simulink model "pi_seqIface"  (R2018b)
settings: Solver=FixedStepDiscrete  StartTime=0.0  StopTime=10.0  RelTol=1e-3
undefined symbols (not defined in the file): boolAliasMember, boolMember, choiceAliasesMember, choiceBuiltInMember, choiceOfFixedSizeSeqOfsMember, choiceOfVarSizeSeqOfsMember, enumAliasMember, enumMember, ia5StringFixedSizeAliasMember, ia5StringFixedSizeMember, ia5StringVarSizeAliasMember, ia5StringVarSizeMember, integerAliasMember, integerMember, octetStringFixedSizeAliasMember, octetStringFixedSizeMember, octetStringVarSizeAliasMember, octetStringVarSizeMember, realAliasMember, realMember
settings Model: Creator=matlab  LastModifiedBy=matlab
settings DataIOCC: SaveOutput=off  SignalLogging=off  SaveTime=off
settings OptimizationCC: DefaultParameterBehavior=Inlined  EnhancedBackFolding=on  PassReuseOutputArgsAs=Individual arguments  OptimizeBlockOrder=speed  DifferentSizesBufferReuse=on  OptimizationCustomize=off
settings DebuggingCC: ParameterTunabilityLossMsg=error
settings SFSimCC: MATLABDynamicMemAlloc=off
settings RTWCC: SystemTargetFile=ert.tlc  TemplateMakefile=ert_default_tmf  PostCodeGenCommand=packNGo(buildInfo);  GenerateReport=on  IncludeHyperlinkInReport=on  LaunchReport=on  GenerateTraceInfo=on  GenerateTraceReport=on  GenerateTraceReportSl=on  GenerateTraceReportSf=on  GenerateTraceReportEml=on
settings CodeAppCC: ForceParamTrailComments=on  IgnoreCustomStorageClasses=off  OperatorAnnotations=on  SimulinkDataObjDesc=on  SFDataObjDesc=on  InsertBlockDesc=on
settings ERTTargetCC: TargetLangStandard=C99 (ISO)  GenerateSampleERTMain=on  InlinedParameterPlacement=NonHierarchical  ERTCustomFileTemplate=example_file_process.tlc

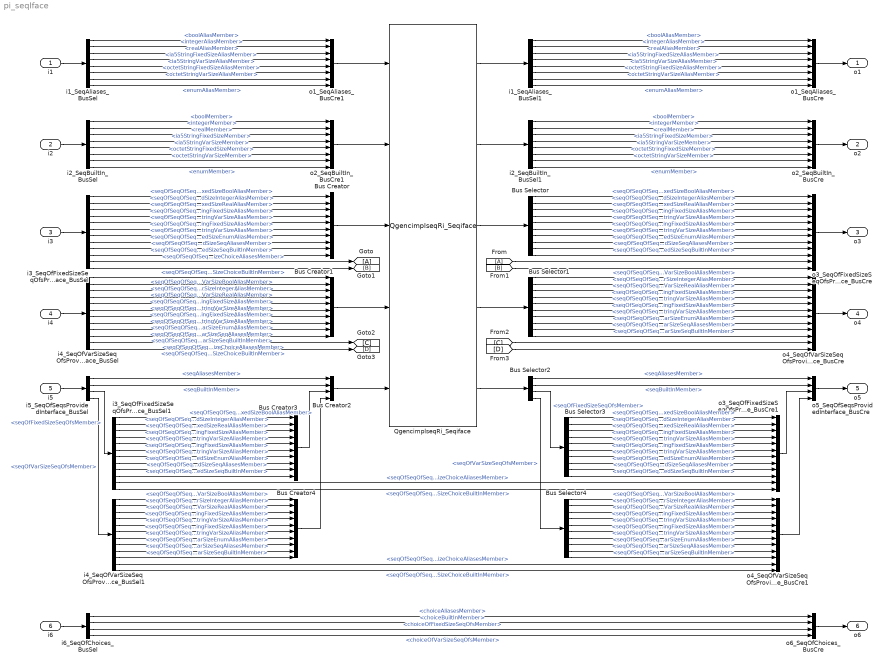
== system pi_seqIface ==
  i1 : Inport  OutDataTypeStr=Bus: SeqAliases  BusOutputAsStruct=on
  i2 : Inport  Port=2  OutDataTypeStr=Bus: SeqBuiltIn  BusOutputAsStruct=on
  i3 : Inport  Port=3  OutDataTypeStr=Bus: SeqOfFixedSizeSeqOfsProvidedInterface  BusOutputAsStruct=on
  i4 : Inport  Port=4  OutDataTypeStr=Bus: SeqOfVarSizeSeqOfsProvidedInterface  BusOutputAsStruct=on
  i5 : Inport  Port=5  OutDataTypeStr=Bus: SeqOfSeqsProvidedInterface  BusOutputAsStruct=on
  i6 : Inport  Port=6  OutDataTypeStr=Bus: SeqOfChoices  BusOutputAsStruct=on
  Bus Creator : BusCreator  Inputs=10  OutDataTypeStr=Bus: SeqOfFixedSizeSeqOfsRequiredInterface  NonVirtualBus=on
  Bus Creator1 : BusCreator  Inputs=10  OutDataTypeStr=Bus: SeqOfVarSizeSeqOfsRequiredInterface  NonVirtualBus=on
  Bus Creator2 : BusCreator  Inputs=4  OutDataTypeStr=Bus: SeqOfSeqsRequiredInterface  NonVirtualBus=on
  Bus Creator3 : BusCreator  Inputs=10  OutDataTypeStr=Bus: SeqOfFixedSizeSeqOfsRequiredInterface  NonVirtualBus=on
  Bus Creator4 : BusCreator  Inputs=10  OutDataTypeStr=Bus: SeqOfVarSizeSeqOfsRequiredInterface  NonVirtualBus=on
  Bus Selector : BusSelector  OutputSignals=seqOfSeqOfSeqOfFixedSizeBoolAliasMember,seqOfSeqOfSeqOfFixedSizeIntegerAliasMember,seqOfSeqOfSeqOfFixedSizeRealAliasMember,seqOfSeqOfSeqOfFixedSizeIA5StringFixedSizeAliasMember,seqOfSeqOfSeqOfFixedSizeIA5StringVarSizeAliasMember,seqOfSeqOfSeqOfFixedSizeOctetStringFixedSizeAliasMember,seqOfSeqOfSeqOfFixedSizeOctetStringVarSizeAliasMember,seqOfSeqOfSeqOfFixedSizeEnumAliasMember,seqOfSeqOfSeqOfFixedSizeSeqAliasesMember,seqOfSeqOfSeqOfFixedSizeSeqBuiltInMember
  Bus Selector1 : BusSelector  OutputSignals=seqOfSeqOfSeqOfVarSizeBoolAliasMember,seqOfSeqOfSeqOfVarSizeIntegerAliasMember,seqOfSeqOfSeqOfVarSizeRealAliasMember,seqOfSeqOfSeqOfVarSizeIA5StringFixedSizeAliasMember,seqOfSeqOfSeqOfVarSizeIA5StringVarSizeAliasMember,seqOfSeqOfSeqOfVarSizeOctetStringFixedSizeAliasMember,seqOfSeqOfSeqOfVarSizeOctetStringVarSizeAliasMember,seqOfSeqOfSeqOfVarSizeEnumAliasMember,seqOfSeqOfSeqOfVarSizeSeqAliasesMember,seqOfSeqOfSeqOfVarSizeSeqBuiltInMember
  Bus Selector2 : BusSelector  OutputSignals=seqAliasesMember,seqBuiltInMember,seqOfFixedSizeSeqOfsMember,seqOfVarSizeSeqOfsMember
  Bus Selector3 : BusSelector  OutputSignals=seqOfSeqOfSeqOfFixedSizeBoolAliasMember,seqOfSeqOfSeqOfFixedSizeIntegerAliasMember,seqOfSeqOfSeqOfFixedSizeRealAliasMember,seqOfSeqOfSeqOfFixedSizeIA5StringFixedSizeAliasMember,seqOfSeqOfSeqOfFixedSizeIA5StringVarSizeAliasMember,seqOfSeqOfSeqOfFixedSizeOctetStringFixedSizeAliasMember,seqOfSeqOfSeqOfFixedSizeOctetStringVarSizeAliasMember,seqOfSeqOfSeqOfFixedSizeEnumAliasMember,seqOfSeqOfSeqOfFixedSizeSeqAliasesMember,seqOfSeqOfSeqOfFixedSizeSeqBuiltInMember
  Bus Selector4 : BusSelector  OutputSignals=seqOfSeqOfSeqOfVarSizeBoolAliasMember,seqOfSeqOfSeqOfVarSizeIntegerAliasMember,seqOfSeqOfSeqOfVarSizeRealAliasMember,seqOfSeqOfSeqOfVarSizeIA5StringFixedSizeAliasMember,seqOfSeqOfSeqOfVarSizeIA5StringVarSizeAliasMember,seqOfSeqOfSeqOfVarSizeOctetStringFixedSizeAliasMember,seqOfSeqOfSeqOfVarSizeOctetStringVarSizeAliasMember,seqOfSeqOfSeqOfVarSizeEnumAliasMember,seqOfSeqOfSeqOfVarSizeSeqAliasesMember,seqOfSeqOfSeqOfVarSizeSeqBuiltInMember
  QgencimplseqRi_Seqiface : S-Function  FunctionName=QgencimplseqRi_Seqiface  SFunctionDeploymentMode=off  EnableBusSupport=off  mask(Legacy Function){SFunctionSpec=void qgencimplseq_RI_ri_seqIface(SeqAliases u1[1], SeqBuiltIn u2[1], SeqOfFixedSizeSeqOfsRequiredInterface u3[1], SeqOfVarSizeSeqOfsRequiredInterface u4[1], SeqOfSeqsRequiredInterface u5[1], SeqAliases y1[1], SeqBuiltIn y2[1], SeqOfFixedSizeSeqOfsRequiredInterface y3[1], SeqOfVarSizeSeqOfsRequiredInterface y4[1], SeqOfSeqsRequiredInterface y5[1]), ShowSpec=off}
      mask prompts: ShowSpec "Display function specification"
      mask help:
      | This block allows you to call the legacy functions specified by the following Legacy Code Tool definition:
      | def.SFunctionName = 'QgencimplseqRi_Seqiface';
      | def.OutputFcnSpec = 'void qgencimplseq_RI_ri_seqIface(SeqAliases u1[1], SeqBuiltIn u2[1], SeqOfFixedSizeSeqOfsRequiredInterface u3[1], SeqOfVarSizeSeqOfsRequiredInterface u4[1], SeqOfSeqsRequiredInterface u5[1], SeqAliases y1[1], SeqBuiltIn y2[1], SeqOfFixedSizeSeqOfsRequiredInterface y3[1], SeqOfVarSizeSeqOfsRequiredInterface y4[1], SeqOfSeqsRequiredInterface y5[1])';
      | def.HeaderFiles = {'qgencimplseq_invoke_ri.h'};
      | def.SourceFiles = {'qgencimplseq_invoke_ri.c'};
      | def.IncPaths = {'..\..\..\dataview\C'};
      mask Help: <p>This block was generated automatically by the Legacy Code Tool. For detailed help on this tool, call<a href="matlab:legacy_code('help')"> legacy_code('help')</a>.</p>
      mask Callback ShowSpec:
      | if strcmp(get_param(gcbh, 'ShowSpec'), 'on')
      |   set_param(gcbh, 'MaskDisplay', sprintf('fprintf(''%s'');', get_param(gcbh, 'SFunctionSpec')));
      | else
      |   set_param(gcbh, 'MaskDisplay', sprintf('fprintf(''%s'');', get_param(gcbh, 'FunctionName')));
      | end
      mask Display: fprintf('QgencimplseqRi_Seqiface');
  i1_SeqAliases_BusSel : BusSelector  OutputSignals=boolAliasMember,integerAliasMember,realAliasMember,ia5StringFixedSizeAliasMember,ia5StringVarSizeAliasMember,octetStringFixedSizeAliasMember,octetStringVarSizeAliasMember,enumAliasMember
  i1_SeqAliases_BusSel1 : BusSelector  OutputSignals=boolAliasMember,integerAliasMember,realAliasMember,ia5StringFixedSizeAliasMember,ia5StringVarSizeAliasMember,octetStringFixedSizeAliasMember,octetStringVarSizeAliasMember,enumAliasMember
  i2_SeqBuiltIn_BusSel : BusSelector  OutputSignals=boolMember,integerMember,realMember,ia5StringFixedSizeMember,ia5StringVarSizeMember,octetStringFixedSizeMember,octetStringVarSizeMember,enumMember
  i2_SeqBuiltIn_BusSel1 : BusSelector  OutputSignals=boolMember,integerMember,realMember,ia5StringFixedSizeMember,ia5StringVarSizeMember,octetStringFixedSizeMember,octetStringVarSizeMember,enumMember
  i3_SeqOfFixedSizeSeqOfsProvidedInterface_BusSel : BusSelector  OutputSignals=seqOfSeqOfSeqOfFixedSizeBoolAliasMember,seqOfSeqOfSeqOfFixedSizeIntegerAliasMember,seqOfSeqOfSeqOfFixedSizeRealAliasMember,seqOfSeqOfSeqOfFixedSizeIA5StringFixedSizeAliasMember,seqOfSeqOfSeqOfFixedSizeIA5StringVarSizeAliasMember,seqOfSeqOfSeqOfFixedSizeOctetStringFixedSizeAliasMember,seqOfSeqOfSeqOfFixedSizeOctetStringVarSizeAliasMember,seqOfSeqOfSeqOfFixedSizeEnumAliasMember,seqOfSeqOfSeqOfFixedSizeSeqAliasesMember,seqOfSeqOfSeqOfFixedSizeSeqBuiltInMember,seqOfSeqOfSeqOfFixedSizeChoiceAliasesMember,seqOfSeqOfSeqOfFixedSizeChoiceBuiltInMember
  i3_SeqOfFixedSizeSeqOfsProvidedInterface_BusSel1 : BusSelector  OutputSignals=seqOfSeqOfSeqOfFixedSizeBoolAliasMember,seqOfSeqOfSeqOfFixedSizeIntegerAliasMember,seqOfSeqOfSeqOfFixedSizeRealAliasMember,seqOfSeqOfSeqOfFixedSizeIA5StringFixedSizeAliasMember,seqOfSeqOfSeqOfFixedSizeIA5StringVarSizeAliasMember,seqOfSeqOfSeqOfFixedSizeOctetStringFixedSizeAliasMember,seqOfSeqOfSeqOfFixedSizeOctetStringVarSizeAliasMember,seqOfSeqOfSeqOfFixedSizeEnumAliasMember,seqOfSeqOfSeqOfFixedSizeSeqAliasesMember,seqOfSeqOfSeqOfFixedSizeSeqBuiltInMember,seqOfSeqOfSeqOfFixedSizeChoiceAliasesMember,seqOfSeqOfSeqOfFixedSizeChoiceBuiltInMember
  i4_SeqOfVarSizeSeqOfsProvidedInterface_BusSel : BusSelector  OutputSignals=seqOfSeqOfSeqOfVarSizeBoolAliasMember,seqOfSeqOfSeqOfVarSizeIntegerAliasMember,seqOfSeqOfSeqOfVarSizeRealAliasMember,seqOfSeqOfSeqOfVarSizeIA5StringFixedSizeAliasMember,seqOfSeqOfSeqOfVarSizeIA5StringVarSizeAliasMember,seqOfSeqOfSeqOfVarSizeOctetStringFixedSizeAliasMember,seqOfSeqOfSeqOfVarSizeOctetStringVarSizeAliasMember,seqOfSeqOfSeqOfVarSizeEnumAliasMember,seqOfSeqOfSeqOfVarSizeSeqAliasesMember,seqOfSeqOfSeqOfVarSizeSeqBuiltInMember,seqOfSeqOfSeqOfVarSizeChoiceAliasesMember,seqOfSeqOfSeqOfVarSizeChoiceBuiltInMember
  i4_SeqOfVarSizeSeqOfsProvidedInterface_BusSel1 : BusSelector  OutputSignals=seqOfSeqOfSeqOfVarSizeBoolAliasMember,seqOfSeqOfSeqOfVarSizeIntegerAliasMember,seqOfSeqOfSeqOfVarSizeRealAliasMember,seqOfSeqOfSeqOfVarSizeIA5StringFixedSizeAliasMember,seqOfSeqOfSeqOfVarSizeIA5StringVarSizeAliasMember,seqOfSeqOfSeqOfVarSizeOctetStringFixedSizeAliasMember,seqOfSeqOfSeqOfVarSizeOctetStringVarSizeAliasMember,seqOfSeqOfSeqOfVarSizeEnumAliasMember,seqOfSeqOfSeqOfVarSizeSeqAliasesMember,seqOfSeqOfSeqOfVarSizeSeqBuiltInMember,seqOfSeqOfSeqOfVarSizeChoiceAliasesMember,seqOfSeqOfSeqOfVarSizeChoiceBuiltInMember
  i5_SeqOfSeqsProvidedInterface_BusSel : BusSelector  OutputSignals=seqAliasesMember,seqBuiltInMember,seqOfFixedSizeSeqOfsMember,seqOfVarSizeSeqOfsMember
  i6_SeqOfChoices_BusSel : BusSelector  OutputSignals=choiceAliasesMember,choiceBuiltInMember,choiceOfFixedSizeSeqOfsMember,choiceOfVarSizeSeqOfsMember
  o1_SeqAliases_BusCre : BusCreator  Inputs=boolAliasMember,integerAliasMember,realAliasMember,ia5StringFixedSizeAliasMember,ia5StringVarSizeAliasMember,octetStringFixedSizeAliasMember,octetStringVarSizeAliasMember,enumAliasMember  OutDataTypeStr=Bus: SeqAliases  NonVirtualBus=on
  o1_SeqAliases_BusCre1 : BusCreator  Inputs=boolAliasMember,integerAliasMember,realAliasMember,ia5StringFixedSizeAliasMember,ia5StringVarSizeAliasMember,octetStringFixedSizeAliasMember,octetStringVarSizeAliasMember,enumAliasMember  OutDataTypeStr=Bus: SeqAliases  NonVirtualBus=on
  o2_SeqBuiltIn_BusCre : BusCreator  Inputs=boolMember,integerMember,realMember,ia5StringFixedSizeMember,ia5StringVarSizeMember,octetStringFixedSizeMember,octetStringVarSizeMember,enumMember  OutDataTypeStr=Bus: SeqBuiltIn  NonVirtualBus=on
  o2_SeqBuiltIn_BusCre1 : BusCreator  Inputs=boolMember,integerMember,realMember,ia5StringFixedSizeMember,ia5StringVarSizeMember,octetStringFixedSizeMember,octetStringVarSizeMember,enumMember  OutDataTypeStr=Bus: SeqBuiltIn  NonVirtualBus=on
  o3_SeqOfFixedSizeSeqOfsProvidedInterface_BusCre : BusCreator  Inputs=seqOfSeqOfSeqOfFixedSizeBoolAliasMember,seqOfSeqOfSeqOfFixedSizeIntegerAliasMember,seqOfSeqOfSeqOfFixedSizeRealAliasMember,seqOfSeqOfSeqOfFixedSizeIA5StringFixedSizeAliasMember,seqOfSeqOfSeqOfFixedSizeIA5StringVarSizeAliasMember,seqOfSeqOfSeqOfFixedSizeOctetStringFixedSizeAliasMember,seqOfSeqOfSeqOfFixedSizeOctetStringVarSizeAliasMember,seqOfSeqOfSeqOfFixedSizeEnumAliasMember,seqOfSeqOfSeqOfFixedSizeSeqAliasesMember,seqOfSeqOfSeqOfFixedSizeSeqBuiltInMember,seqOfSeqOfSeqOfFixedSizeChoiceAliasesMember,seqOfSeqOfSeqOfFixedSizeChoiceBuiltInMember  OutDataTypeStr=Bus: SeqOfFixedSizeSeqOfsProvidedInterface  NonVirtualBus=on
  o3_SeqOfFixedSizeSeqOfsProvidedInterface_BusCre1 : BusCreator  Inputs=12  OutDataTypeStr=Bus: SeqOfFixedSizeSeqOfsProvidedInterface  NonVirtualBus=on
  o4_SeqOfVarSizeSeqOfsProvidedInterface_BusCre : BusCreator  Inputs=seqOfSeqOfSeqOfVarSizeBoolAliasMember,seqOfSeqOfSeqOfVarSizeIntegerAliasMember,seqOfSeqOfSeqOfVarSizeRealAliasMember,seqOfSeqOfSeqOfVarSizeIA5StringFixedSizeAliasMember,seqOfSeqOfSeqOfVarSizeIA5StringVarSizeAliasMember,seqOfSeqOfSeqOfVarSizeOctetStringFixedSizeAliasMember,seqOfSeqOfSeqOfVarSizeOctetStringVarSizeAliasMember,seqOfSeqOfSeqOfVarSizeEnumAliasMember,seqOfSeqOfSeqOfVarSizeSeqAliasesMember,seqOfSeqOfSeqOfVarSizeSeqBuiltInMember,seqOfSeqOfSeqOfVarSizeChoiceAliasesMember,seqOfSeqOfSeqOfVarSizeChoiceBuiltInMember  OutDataTypeStr=Bus: SeqOfVarSizeSeqOfsProvidedInterface  NonVirtualBus=on
  o4_SeqOfVarSizeSeqOfsProvidedInterface_BusCre1 : BusCreator  Inputs=seqOfSeqOfSeqOfVarSizeBoolAliasMember,seqOfSeqOfSeqOfVarSizeIntegerAliasMember,seqOfSeqOfSeqOfVarSizeRealAliasMember,seqOfSeqOfSeqOfVarSizeIA5StringFixedSizeAliasMember,seqOfSeqOfSeqOfVarSizeIA5StringVarSizeAliasMember,seqOfSeqOfSeqOfVarSizeOctetStringFixedSizeAliasMember,seqOfSeqOfSeqOfVarSizeOctetStringVarSizeAliasMember,seqOfSeqOfSeqOfVarSizeEnumAliasMember,seqOfSeqOfSeqOfVarSizeSeqAliasesMember,seqOfSeqOfSeqOfVarSizeSeqBuiltInMember,seqOfSeqOfSeqOfVarSizeChoiceAliasesMember,seqOfSeqOfSeqOfVarSizeChoiceBuiltInMember  OutDataTypeStr=Bus: SeqOfVarSizeSeqOfsProvidedInterface  NonVirtualBus=on
  o5_SeqOfSeqsProvidedInterface_BusCre : BusCreator  Inputs=4  OutDataTypeStr=Bus: SeqOfSeqsProvidedInterface  NonVirtualBus=on
  o6_SeqOfChoices_BusCre : BusCreator  Inputs=choiceAliasesMember,choiceBuiltInMember,choiceOfFixedSizeSeqOfsMember,choiceOfVarSizeSeqOfsMember  OutDataTypeStr=Bus: SeqOfChoices  NonVirtualBus=on
  o1 : Outport  OutDataTypeStr=Bus: SeqAliases  BusOutputAsStruct=on
  o2 : Outport  Port=2  OutDataTypeStr=Bus: SeqBuiltIn  BusOutputAsStruct=on
  o3 : Outport  Port=3  OutDataTypeStr=Bus: SeqOfFixedSizeSeqOfsProvidedInterface  BusOutputAsStruct=on
  o4 : Outport  Port=4  OutDataTypeStr=Bus: SeqOfVarSizeSeqOfsProvidedInterface  BusOutputAsStruct=on
  o5 : Outport  Port=5  OutDataTypeStr=Bus: SeqOfSeqsProvidedInterface  BusOutputAsStruct=on
  o6 : Outport  Port=6  OutDataTypeStr=Bus: SeqOfChoices  BusOutputAsStruct=on
  wires:
  i1/1 -> i1_SeqAliases_BusSel/1
  i2/1 -> i2_SeqBuiltIn_BusSel/1
  i3/1 -> i3_SeqOfFixedSizeSeqOfsProvidedInterface_BusSel/1
  i4/1 -> i4_SeqOfVarSizeSeqOfsProvidedInterface_BusSel/1
  i5/1 -> i5_SeqOfSeqsProvidedInterface_BusSel/1
  i6/1 -> i6_SeqOfChoices_BusSel/1
  o1_SeqAliases_BusCre/1 -> o1/1
  o2_SeqBuiltIn_BusCre/1 -> o2/1
  o3_SeqOfFixedSizeSeqOfsProvidedInterface_BusCre/1 -> o3/1
  o4_SeqOfVarSizeSeqOfsProvidedInterface_BusCre/1 -> o4/1
  o5_SeqOfSeqsProvidedInterface_BusCre/1 -> o5/1
  o6_SeqOfChoices_BusCre/1 -> o6/1
  o1_SeqAliases_BusCre1/1 -> QgencimplseqRi_Seqiface/1
  i1_SeqAliases_BusSel/1 -> o1_SeqAliases_BusCre1/1  "<boolAliasMember>"
  i1_SeqAliases_BusSel/2 -> o1_SeqAliases_BusCre1/2  "<integerAliasMember>"
  i1_SeqAliases_BusSel/3 -> o1_SeqAliases_BusCre1/3  "<realAliasMember>"
  i1_SeqAliases_BusSel/4 -> o1_SeqAliases_BusCre1/4  "<ia5StringFixedSizeAliasMember>"
  i1_SeqAliases_BusSel/5 -> o1_SeqAliases_BusCre1/5  "<ia5StringVarSizeAliasMember>"
  i1_SeqAliases_BusSel/6 -> o1_SeqAliases_BusCre1/6  "<octetStringFixedSizeAliasMember>"
  i1_SeqAliases_BusSel/7 -> o1_SeqAliases_BusCre1/7  "<octetStringVarSizeAliasMember>"
  i1_SeqAliases_BusSel/8 -> o1_SeqAliases_BusCre1/8  "<enumAliasMember>"
  i2_SeqBuiltIn_BusSel/1 -> o2_SeqBuiltIn_BusCre1/1  "<boolMember>"
  i2_SeqBuiltIn_BusSel/2 -> o2_SeqBuiltIn_BusCre1/2  "<integerMember>"
  i2_SeqBuiltIn_BusSel/3 -> o2_SeqBuiltIn_BusCre1/3  "<realMember>"
  i2_SeqBuiltIn_BusSel/4 -> o2_SeqBuiltIn_BusCre1/4  "<ia5StringFixedSizeMember>"
  i2_SeqBuiltIn_BusSel/5 -> o2_SeqBuiltIn_BusCre1/5  "<ia5StringVarSizeMember>"
  i2_SeqBuiltIn_BusSel/6 -> o2_SeqBuiltIn_BusCre1/6  "<octetStringFixedSizeMember>"
  i2_SeqBuiltIn_BusSel/7 -> o2_SeqBuiltIn_BusCre1/7  "<octetStringVarSizeMember>"
  i2_SeqBuiltIn_BusSel/8 -> o2_SeqBuiltIn_BusCre1/8  "<enumMember>"
  o2_SeqBuiltIn_BusCre1/1 -> QgencimplseqRi_Seqiface/2
  QgencimplseqRi_Seqiface/1 -> i1_SeqAliases_BusSel1/1
  i1_SeqAliases_BusSel1/1 -> o1_SeqAliases_BusCre/1  "<boolAliasMember>"
  i1_SeqAliases_BusSel1/2 -> o1_SeqAliases_BusCre/2  "<integerAliasMember>"
  i1_SeqAliases_BusSel1/3 -> o1_SeqAliases_BusCre/3  "<realAliasMember>"
  i1_SeqAliases_BusSel1/4 -> o1_SeqAliases_BusCre/4  "<ia5StringFixedSizeAliasMember>"
  i1_SeqAliases_BusSel1/5 -> o1_SeqAliases_BusCre/5  "<ia5StringVarSizeAliasMember>"
  i1_SeqAliases_BusSel1/6 -> o1_SeqAliases_BusCre/6  "<octetStringFixedSizeAliasMember>"
  i1_SeqAliases_BusSel1/7 -> o1_SeqAliases_BusCre/7  "<octetStringVarSizeAliasMember>"
  i1_SeqAliases_BusSel1/8 -> o1_SeqAliases_BusCre/8  "<enumAliasMember>"
  QgencimplseqRi_Seqiface/2 -> i2_SeqBuiltIn_BusSel1/1
  i2_SeqBuiltIn_BusSel1/1 -> o2_SeqBuiltIn_BusCre/1  "<boolMember>"
  i2_SeqBuiltIn_BusSel1/2 -> o2_SeqBuiltIn_BusCre/2  "<integerMember>"
  i2_SeqBuiltIn_BusSel1/3 -> o2_SeqBuiltIn_BusCre/3  "<realMember>"
  i2_SeqBuiltIn_BusSel1/4 -> o2_SeqBuiltIn_BusCre/4  "<ia5StringFixedSizeMember>"
  i2_SeqBuiltIn_BusSel1/5 -> o2_SeqBuiltIn_BusCre/5  "<ia5StringVarSizeMember>"
  i2_SeqBuiltIn_BusSel1/6 -> o2_SeqBuiltIn_BusCre/6  "<octetStringFixedSizeMember>"
  i2_SeqBuiltIn_BusSel1/7 -> o2_SeqBuiltIn_BusCre/7  "<octetStringVarSizeMember>"
  i2_SeqBuiltIn_BusSel1/8 -> o2_SeqBuiltIn_BusCre/8  "<enumMember>"
  Bus Selector/1 -> o3_SeqOfFixedSizeSeqOfsProvidedInterface_BusCre/1  "<seqOfSeqOfSeqOfFixedSizeBoolAliasMember>"
  Bus Selector/2 -> o3_SeqOfFixedSizeSeqOfsProvidedInterface_BusCre/2  "<seqOfSeqOfSeqOfFixedSizeIntegerAliasMember>"
  Bus Selector/3 -> o3_SeqOfFixedSizeSeqOfsProvidedInterface_BusCre/3  "<seqOfSeqOfSeqOfFixedSizeRealAliasMember>"
  Bus Selector/4 -> o3_SeqOfFixedSizeSeqOfsProvidedInterface_BusCre/4  "<seqOfSeqOfSeqOfFixedSizeIA5StringFixedSizeAliasMember>"
  Bus Selector/5 -> o3_SeqOfFixedSizeSeqOfsProvidedInterface_BusCre/5  "<seqOfSeqOfSeqOfFixedSizeIA5StringVarSizeAliasMember>"
  Bus Selector/6 -> o3_SeqOfFixedSizeSeqOfsProvidedInterface_BusCre/6  "<seqOfSeqOfSeqOfFixedSizeOctetStringFixedSizeAliasMember>"
  Bus Selector/7 -> o3_SeqOfFixedSizeSeqOfsProvidedInterface_BusCre/7  "<seqOfSeqOfSeqOfFixedSizeOctetStringVarSizeAliasMember>"
  Bus Selector/8 -> o3_SeqOfFixedSizeSeqOfsProvidedInterface_BusCre/8  "<seqOfSeqOfSeqOfFixedSizeEnumAliasMember>"
  Bus Selector/9 -> o3_SeqOfFixedSizeSeqOfsProvidedInterface_BusCre/9  "<seqOfSeqOfSeqOfFixedSizeSeqAliasesMember>"
  Bus Selector/10 -> o3_SeqOfFixedSizeSeqOfsProvidedInterface_BusCre/10  "<seqOfSeqOfSeqOfFixedSizeSeqBuiltInMember>"
  [A] -> o3_SeqOfFixedSizeSeqOfsProvidedInterface_BusCre/11
  [B] -> o3_SeqOfFixedSizeSeqOfsProvidedInterface_BusCre/12
  Bus Selector1/2 -> o4_SeqOfVarSizeSeqOfsProvidedInterface_BusCre/2  "<seqOfSeqOfSeqOfVarSizeIntegerAliasMember>"
  Bus Selector1/3 -> o4_SeqOfVarSizeSeqOfsProvidedInterface_BusCre/3  "<seqOfSeqOfSeqOfVarSizeRealAliasMember>"
  Bus Selector1/4 -> o4_SeqOfVarSizeSeqOfsProvidedInterface_BusCre/4  "<seqOfSeqOfSeqOfVarSizeIA5StringFixedSizeAliasMember>"
  Bus Selector1/5 -> o4_SeqOfVarSizeSeqOfsProvidedInterface_BusCre/5  "<seqOfSeqOfSeqOfVarSizeIA5StringVarSizeAliasMember>"
  Bus Selector1/6 -> o4_SeqOfVarSizeSeqOfsProvidedInterface_BusCre/6  "<seqOfSeqOfSeqOfVarSizeOctetStringFixedSizeAliasMember>"
  Bus Selector1/7 -> o4_SeqOfVarSizeSeqOfsProvidedInterface_BusCre/7  "<seqOfSeqOfSeqOfVarSizeOctetStringVarSizeAliasMember>"
  Bus Selector1/8 -> o4_SeqOfVarSizeSeqOfsProvidedInterface_BusCre/8  "<seqOfSeqOfSeqOfVarSizeEnumAliasMember>"
  Bus Selector1/9 -> o4_SeqOfVarSizeSeqOfsProvidedInterface_BusCre/9  "<seqOfSeqOfSeqOfVarSizeSeqAliasesMember>"
  Bus Selector1/10 -> o4_SeqOfVarSizeSeqOfsProvidedInterface_BusCre/10  "<seqOfSeqOfSeqOfVarSizeSeqBuiltInMember>"
  Bus Selector1/1 -> o4_SeqOfVarSizeSeqOfsProvidedInterface_BusCre/1  "<seqOfSeqOfSeqOfVarSizeBoolAliasMember>"
  QgencimplseqRi_Seqiface/3 -> Bus Selector/1
  [C] -> o4_SeqOfVarSizeSeqOfsProvidedInterface_BusCre/11
  [D] -> o4_SeqOfVarSizeSeqOfsProvidedInterface_BusCre/12
  i3_SeqOfFixedSizeSeqOfsProvidedInterface_BusSel/1 -> Bus Creator/1  "<seqOfSeqOfSeqOfFixedSizeBoolAliasMember>"
  i3_SeqOfFixedSizeSeqOfsProvidedInterface_BusSel/2 -> Bus Creator/2  "<seqOfSeqOfSeqOfFixedSizeIntegerAliasMember>"
  i3_SeqOfFixedSizeSeqOfsProvidedInterface_BusSel/3 -> Bus Creator/3  "<seqOfSeqOfSeqOfFixedSizeRealAliasMember>"
  i3_SeqOfFixedSizeSeqOfsProvidedInterface_BusSel/4 -> Bus Creator/4  "<seqOfSeqOfSeqOfFixedSizeIA5StringFixedSizeAliasMember>"
  i3_SeqOfFixedSizeSeqOfsProvidedInterface_BusSel/5 -> Bus Creator/5  "<seqOfSeqOfSeqOfFixedSizeIA5StringVarSizeAliasMember>"
  i3_SeqOfFixedSizeSeqOfsProvidedInterface_BusSel/6 -> Bus Creator/6  "<seqOfSeqOfSeqOfFixedSizeOctetStringFixedSizeAliasMember>"
  i3_SeqOfFixedSizeSeqOfsProvidedInterface_BusSel/7 -> Bus Creator/7  "<seqOfSeqOfSeqOfFixedSizeOctetStringVarSizeAliasMember>"
  i3_SeqOfFixedSizeSeqOfsProvidedInterface_BusSel/8 -> Bus Creator/8  "<seqOfSeqOfSeqOfFixedSizeEnumAliasMember>"
  i3_SeqOfFixedSizeSeqOfsProvidedInterface_BusSel/9 -> Bus Creator/9  "<seqOfSeqOfSeqOfFixedSizeSeqAliasesMember>"
  i3_SeqOfFixedSizeSeqOfsProvidedInterface_BusSel/10 -> Bus Creator/10  "<seqOfSeqOfSeqOfFixedSizeSeqBuiltInMember>"
  i3_SeqOfFixedSizeSeqOfsProvidedInterface_BusSel/11 -> [A]  "<seqOfSeqOfSeqOfFixedSizeChoiceAliasesMember>"
  i3_SeqOfFixedSizeSeqOfsProvidedInterface_BusSel/12 -> [B]  "<seqOfSeqOfSeqOfFixedSizeChoiceBuiltInMember>"
  Bus Creator/1 -> QgencimplseqRi_Seqiface/3
  i4_SeqOfVarSizeSeqOfsProvidedInterface_BusSel/1 -> Bus Creator1/1  "<seqOfSeqOfSeqOfVarSizeBoolAliasMember>"
  i4_SeqOfVarSizeSeqOfsProvidedInterface_BusSel/2 -> Bus Creator1/2  "<seqOfSeqOfSeqOfVarSizeIntegerAliasMember>"
  i4_SeqOfVarSizeSeqOfsProvidedInterface_BusSel/3 -> Bus Creator1/3  "<seqOfSeqOfSeqOfVarSizeRealAliasMember>"
  i4_SeqOfVarSizeSeqOfsProvidedInterface_BusSel/4 -> Bus Creator1/4  "<seqOfSeqOfSeqOfVarSizeIA5StringFixedSizeAliasMember>"
  i4_SeqOfVarSizeSeqOfsProvidedInterface_BusSel/5 -> Bus Creator1/5  "<seqOfSeqOfSeqOfVarSizeIA5StringVarSizeAliasMember>"
  i4_SeqOfVarSizeSeqOfsProvidedInterface_BusSel/6 -> Bus Creator1/6  "<seqOfSeqOfSeqOfVarSizeOctetStringFixedSizeAliasMember>"
  i4_SeqOfVarSizeSeqOfsProvidedInterface_BusSel/7 -> Bus Creator1/7  "<seqOfSeqOfSeqOfVarSizeOctetStringVarSizeAliasMember>"
  i4_SeqOfVarSizeSeqOfsProvidedInterface_BusSel/8 -> Bus Creator1/8  "<seqOfSeqOfSeqOfVarSizeEnumAliasMember>"
  i4_SeqOfVarSizeSeqOfsProvidedInterface_BusSel/9 -> Bus Creator1/9  "<seqOfSeqOfSeqOfVarSizeSeqAliasesMember>"
  i4_SeqOfVarSizeSeqOfsProvidedInterface_BusSel/10 -> Bus Creator1/10  "<seqOfSeqOfSeqOfVarSizeSeqBuiltInMember>"
  Bus Creator1/1 -> QgencimplseqRi_Seqiface/4
  QgencimplseqRi_Seqiface/4 -> Bus Selector1/1
  i6_SeqOfChoices_BusSel/1 -> o6_SeqOfChoices_BusCre/1  "<choiceAliasesMember>"
  i6_SeqOfChoices_BusSel/2 -> o6_SeqOfChoices_BusCre/2  "<choiceBuiltInMember>"
  i6_SeqOfChoices_BusSel/3 -> o6_SeqOfChoices_BusCre/3  "<choiceOfFixedSizeSeqOfsMember>"
  i6_SeqOfChoices_BusSel/4 -> o6_SeqOfChoices_BusCre/4  "<choiceOfVarSizeSeqOfsMember>"
  QgencimplseqRi_Seqiface/5 -> Bus Selector2/1
  Bus Creator2/1 -> QgencimplseqRi_Seqiface/5
  i5_SeqOfSeqsProvidedInterface_BusSel/1 -> Bus Creator2/1  "<seqAliasesMember>"
  i5_SeqOfSeqsProvidedInterface_BusSel/2 -> Bus Creator2/2  "<seqBuiltInMember>"
  i4_SeqOfVarSizeSeqOfsProvidedInterface_BusSel/11 -> [C]  "<seqOfSeqOfSeqOfVarSizeChoiceAliasesMember>"
  i4_SeqOfVarSizeSeqOfsProvidedInterface_BusSel/12 -> [D]  "<seqOfSeqOfSeqOfVarSizeChoiceBuiltInMember>"
  i4_SeqOfVarSizeSeqOfsProvidedInterface_BusSel1/7 -> Bus Creator4/7  "<seqOfSeqOfSeqOfVarSizeOctetStringVarSizeAliasMember>"
  i4_SeqOfVarSizeSeqOfsProvidedInterface_BusSel1/9 -> Bus Creator4/9  "<seqOfSeqOfSeqOfVarSizeSeqAliasesMember>"
  i4_SeqOfVarSizeSeqOfsProvidedInterface_BusSel1/4 -> Bus Creator4/4  "<seqOfSeqOfSeqOfVarSizeIA5StringFixedSizeAliasMember>"
  i4_SeqOfVarSizeSeqOfsProvidedInterface_BusSel1/2 -> Bus Creator4/2  "<seqOfSeqOfSeqOfVarSizeIntegerAliasMember>"
  i4_SeqOfVarSizeSeqOfsProvidedInterface_BusSel1/5 -> Bus Creator4/5  "<seqOfSeqOfSeqOfVarSizeIA5StringVarSizeAliasMember>"
  i5_SeqOfSeqsProvidedInterface_BusSel/3 -> i3_SeqOfFixedSizeSeqOfsProvidedInterface_BusSel1/1  "<seqOfFixedSizeSeqOfsMember>"
  i3_SeqOfFixedSizeSeqOfsProvidedInterface_BusSel1/7 -> Bus Creator3/7  "<seqOfSeqOfSeqOfFixedSizeOctetStringVarSizeAliasMember>"
  i3_SeqOfFixedSizeSeqOfsProvidedInterface_BusSel1/5 -> Bus Creator3/5  "<seqOfSeqOfSeqOfFixedSizeIA5StringVarSizeAliasMember>"
  i4_SeqOfVarSizeSeqOfsProvidedInterface_BusSel1/11 -> o4_SeqOfVarSizeSeqOfsProvidedInterface_BusCre1/11  "<seqOfSeqOfSeqOfVarSizeChoiceAliasesMember>"
  i4_SeqOfVarSizeSeqOfsProvidedInterface_BusSel1/10 -> Bus Creator4/10  "<seqOfSeqOfSeqOfVarSizeSeqBuiltInMember>"
  i4_SeqOfVarSizeSeqOfsProvidedInterface_BusSel1/12 -> o4_SeqOfVarSizeSeqOfsProvidedInterface_BusCre1/12  "<seqOfSeqOfSeqOfVarSizeChoiceBuiltInMember>"
  i3_SeqOfFixedSizeSeqOfsProvidedInterface_BusSel1/10 -> Bus Creator3/10  "<seqOfSeqOfSeqOfFixedSizeSeqBuiltInMember>"
  i3_SeqOfFixedSizeSeqOfsProvidedInterface_BusSel1/12 -> o3_SeqOfFixedSizeSeqOfsProvidedInterface_BusCre1/12  "<seqOfSeqOfSeqOfFixedSizeChoiceBuiltInMember>"
  i4_SeqOfVarSizeSeqOfsProvidedInterface_BusSel1/3 -> Bus Creator4/3  "<seqOfSeqOfSeqOfVarSizeRealAliasMember>"
  i3_SeqOfFixedSizeSeqOfsProvidedInterface_BusSel1/2 -> Bus Creator3/2  "<seqOfSeqOfSeqOfFixedSizeIntegerAliasMember>"
  i3_SeqOfFixedSizeSeqOfsProvidedInterface_BusSel1/1 -> Bus Creator3/1  "<seqOfSeqOfSeqOfFixedSizeBoolAliasMember>"
  i5_SeqOfSeqsProvidedInterface_BusSel/4 -> i4_SeqOfVarSizeSeqOfsProvidedInterface_BusSel1/1  "<seqOfVarSizeSeqOfsMember>"
  i4_SeqOfVarSizeSeqOfsProvidedInterface_BusSel1/1 -> Bus Creator4/1  "<seqOfSeqOfSeqOfVarSizeBoolAliasMember>"
  i4_SeqOfVarSizeSeqOfsProvidedInterface_BusSel1/6 -> Bus Creator4/6  "<seqOfSeqOfSeqOfVarSizeOctetStringFixedSizeAliasMember>"
  i3_SeqOfFixedSizeSeqOfsProvidedInterface_BusSel1/8 -> Bus Creator3/8  "<seqOfSeqOfSeqOfFixedSizeEnumAliasMember>"
  i3_SeqOfFixedSizeSeqOfsProvidedInterface_BusSel1/3 -> Bus Creator3/3  "<seqOfSeqOfSeqOfFixedSizeRealAliasMember>"
  i3_SeqOfFixedSizeSeqOfsProvidedInterface_BusSel1/4 -> Bus Creator3/4  "<seqOfSeqOfSeqOfFixedSizeIA5StringFixedSizeAliasMember>"
  i3_SeqOfFixedSizeSeqOfsProvidedInterface_BusSel1/9 -> Bus Creator3/9  "<seqOfSeqOfSeqOfFixedSizeSeqAliasesMember>"
  i4_SeqOfVarSizeSeqOfsProvidedInterface_BusSel1/8 -> Bus Creator4/8  "<seqOfSeqOfSeqOfVarSizeEnumAliasMember>"
  i3_SeqOfFixedSizeSeqOfsProvidedInterface_BusSel1/11 -> o3_SeqOfFixedSizeSeqOfsProvidedInterface_BusCre1/11  "<seqOfSeqOfSeqOfFixedSizeChoiceAliasesMember>"
  i3_SeqOfFixedSizeSeqOfsProvidedInterface_BusSel1/6 -> Bus Creator3/6  "<seqOfSeqOfSeqOfFixedSizeOctetStringFixedSizeAliasMember>"
  Bus Creator3/1 -> Bus Creator2/3
  Bus Creator4/1 -> Bus Creator2/4
  Bus Selector2/1 -> o5_SeqOfSeqsProvidedInterface_BusCre/1  "<seqAliasesMember>"
  Bus Selector2/2 -> o5_SeqOfSeqsProvidedInterface_BusCre/2  "<seqBuiltInMember>"
  Bus Selector3/10 -> o3_SeqOfFixedSizeSeqOfsProvidedInterface_BusCre1/10  "<seqOfSeqOfSeqOfFixedSizeSeqBuiltInMember>"
  Bus Selector3/2 -> o3_SeqOfFixedSizeSeqOfsProvidedInterface_BusCre1/2  "<seqOfSeqOfSeqOfFixedSizeIntegerAliasMember>"
  Bus Selector3/8 -> o3_SeqOfFixedSizeSeqOfsProvidedInterface_BusCre1/8  "<seqOfSeqOfSeqOfFixedSizeEnumAliasMember>"
  Bus Selector3/5 -> o3_SeqOfFixedSizeSeqOfsProvidedInterface_BusCre1/5  "<seqOfSeqOfSeqOfFixedSizeIA5StringVarSizeAliasMember>"
  Bus Selector3/9 -> o3_SeqOfFixedSizeSeqOfsProvidedInterface_BusCre1/9  "<seqOfSeqOfSeqOfFixedSizeSeqAliasesMember>"
  Bus Selector3/3 -> o3_SeqOfFixedSizeSeqOfsProvidedInterface_BusCre1/3  "<seqOfSeqOfSeqOfFixedSizeRealAliasMember>"
  Bus Selector3/4 -> o3_SeqOfFixedSizeSeqOfsProvidedInterface_BusCre1/4  "<seqOfSeqOfSeqOfFixedSizeIA5StringFixedSizeAliasMember>"
  Bus Selector3/7 -> o3_SeqOfFixedSizeSeqOfsProvidedInterface_BusCre1/7  "<seqOfSeqOfSeqOfFixedSizeOctetStringVarSizeAliasMember>"
  Bus Selector3/1 -> o3_SeqOfFixedSizeSeqOfsProvidedInterface_BusCre1/1  "<seqOfSeqOfSeqOfFixedSizeBoolAliasMember>"
  Bus Selector2/3 -> Bus Selector3/1  "<seqOfFixedSizeSeqOfsMember>"
  Bus Selector3/6 -> o3_SeqOfFixedSizeSeqOfsProvidedInterface_BusCre1/6  "<seqOfSeqOfSeqOfFixedSizeOctetStringFixedSizeAliasMember>"
  Bus Selector4/1 -> o4_SeqOfVarSizeSeqOfsProvidedInterface_BusCre1/1  "<seqOfSeqOfSeqOfVarSizeBoolAliasMember>"
  Bus Selector4/9 -> o4_SeqOfVarSizeSeqOfsProvidedInterface_BusCre1/9  "<seqOfSeqOfSeqOfVarSizeSeqAliasesMember>"
  Bus Selector4/10 -> o4_SeqOfVarSizeSeqOfsProvidedInterface_BusCre1/10  "<seqOfSeqOfSeqOfVarSizeSeqBuiltInMember>"
  Bus Selector4/8 -> o4_SeqOfVarSizeSeqOfsProvidedInterface_BusCre1/8  "<seqOfSeqOfSeqOfVarSizeEnumAliasMember>"
  Bus Selector4/4 -> o4_SeqOfVarSizeSeqOfsProvidedInterface_BusCre1/4  "<seqOfSeqOfSeqOfVarSizeIA5StringFixedSizeAliasMember>"
  Bus Selector4/6 -> o4_SeqOfVarSizeSeqOfsProvidedInterface_BusCre1/6  "<seqOfSeqOfSeqOfVarSizeOctetStringFixedSizeAliasMember>"
  Bus Selector4/5 -> o4_SeqOfVarSizeSeqOfsProvidedInterface_BusCre1/5  "<seqOfSeqOfSeqOfVarSizeIA5StringVarSizeAliasMember>"
  Bus Selector4/3 -> o4_SeqOfVarSizeSeqOfsProvidedInterface_BusCre1/3  "<seqOfSeqOfSeqOfVarSizeRealAliasMember>"
  Bus Selector4/2 -> o4_SeqOfVarSizeSeqOfsProvidedInterface_BusCre1/2  "<seqOfSeqOfSeqOfVarSizeIntegerAliasMember>"
  Bus Selector2/4 -> Bus Selector4/1  "<seqOfVarSizeSeqOfsMember>"
  Bus Selector4/7 -> o4_SeqOfVarSizeSeqOfsProvidedInterface_BusCre1/7  "<seqOfSeqOfSeqOfVarSizeOctetStringVarSizeAliasMember>"
  o3_SeqOfFixedSizeSeqOfsProvidedInterface_BusCre1/1 -> o5_SeqOfSeqsProvidedInterface_BusCre/3
  o4_SeqOfVarSizeSeqOfsProvidedInterface_BusCre1/1 -> o5_SeqOfSeqsProvidedInterface_BusCre/4
